simulink model "car_park_simulation"  (R2023b)
settings: Solver=VariableStepAuto  StartTime=0.0  StopTime=inf  RelTol=1e-3
libraries: simulink_extras x8, simulink x2
settings Model: Creator=abdul  LastModifiedBy=abdul

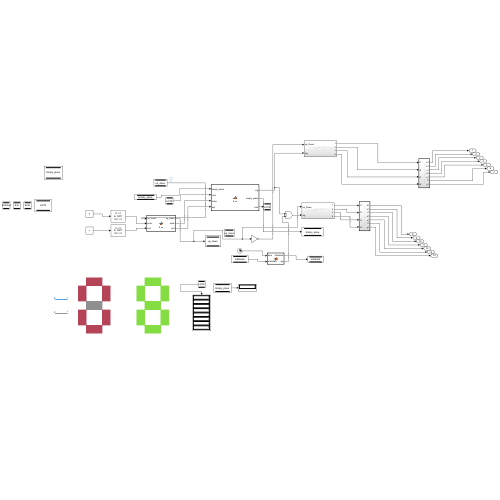
[thumbnail: Simulink's stored preview of the top-level diagram]
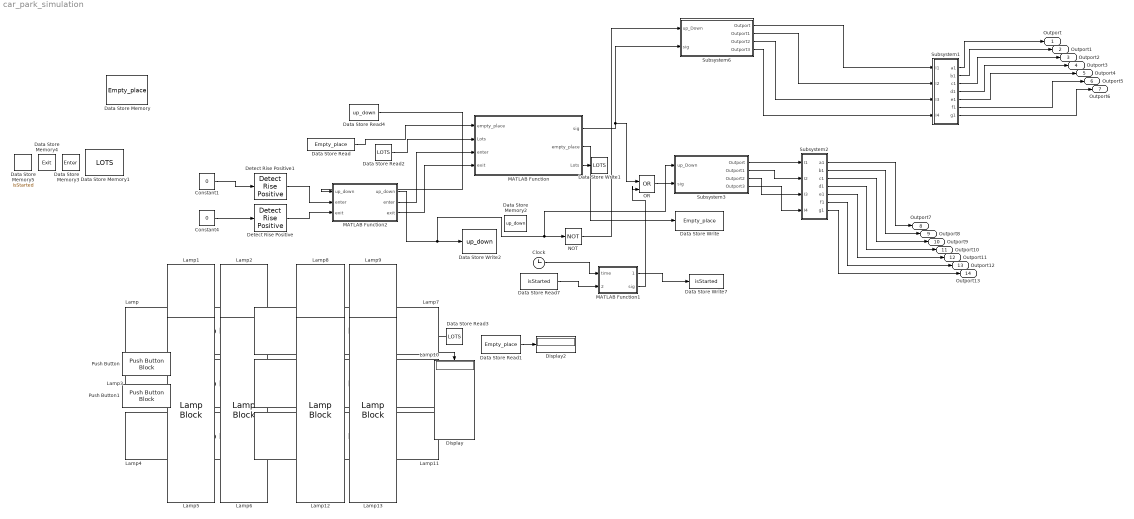
== system car_park_simulation ==
  Clock : Clock
  Constant1 : Constant  Value=0
  Constant4 : Constant  Value=0
  Data Store Memory : DataStoreMemory  DataStoreName=Empty_place  WriteAfterWriteMsg=warning  InitialValue=8  ShowAdditionalParam=off  OutDataTypeStr=double
  Data Store Memory1 : DataStoreMemory  DataStoreName=LOTS  WriteAfterWriteMsg=warning  InitialValue=[0,0,0,0,0,0,0,0]  ShowAdditionalParam=off
  Data Store Memory2 : DataStoreMemory  DataStoreName=up_down  WriteAfterWriteMsg=warning  ShowAdditionalParam=off
  Data Store Memory3 : DataStoreMemory  DataStoreName=Enter  WriteAfterWriteMsg=warning  ShowAdditionalParam=off
  Data Store Memory4 : DataStoreMemory  DataStoreName=Exit  WriteAfterWriteMsg=warning  ShowAdditionalParam=off
  Data Store Memory5 : DataStoreMemory  DataStoreName=isStarted  WriteAfterWriteMsg=warning  ShowAdditionalParam=off
  Data Store Read : DataStoreRead  DataStoreName=Empty_place  IndexOptions=Index vector (dialog)  Indices=1  OutputSizes=1
  Data Store Read1 : DataStoreRead  DataStoreName=Empty_place  IndexOptions=Index vector (dialog)  Indices=1  OutputSizes=1
  Data Store Read2 : DataStoreRead  DataStoreName=LOTS  IndexOptions=Index vector (dialog)  Indices=1  OutputSizes=1
  Data Store Read3 : DataStoreRead  DataStoreName=LOTS  IndexOptions=Index vector (dialog)  Indices=1  OutputSizes=1
  Data Store Read4 : DataStoreRead  DataStoreName=up_down  IndexOptions=Index vector (dialog)  Indices=1  OutputSizes=1
  Data Store Read7 : DataStoreRead  DataStoreName=isStarted  IndexOptions=Index vector (dialog)  Indices=1  OutputSizes=1
  Data Store Write : DataStoreWrite  DataStoreName=Empty_place  IndexOptions=Index vector (dialog)  Indices=1  OutputSizes=1
  Data Store Write1 : DataStoreWrite  DataStoreName=LOTS  IndexOptions=Index vector (dialog)  Indices=1  OutputSizes=1
  Data Store Write2 : DataStoreWrite  DataStoreName=up_down  IndexOptions=Index vector (dialog)  Indices=1  OutputSizes=1
  Data Store Write7 : DataStoreWrite  DataStoreName=isStarted  IndexOptions=Index vector (dialog)  Indices=1  OutputSizes=1
  Detect Rise Positive : simulink/Logic and Bit Operations/Detect Rise Positive  vinit=0  OutDataTypeStr=boolean
  Detect Rise Positive1 : simulink/Logic and Bit Operations/Detect Rise Positive  vinit=0  OutDataTypeStr=boolean
  Display : Display
  Display2 : Display
  Lamp{,1..13} (14 alike) : LampBlock  LabelPosition=Hide  Icon=Rectangle
  MATLAB Function : MATLAB Function  TreatAsAtomicUnit=on
  MATLAB Function1 : MATLAB Function  TreatAsAtomicUnit=on
  MATLAB Function2 : MATLAB Function  TreatAsAtomicUnit=on
  NOT : Logic  Operator=NOT  IconShape=distinctive  AllPortsSameDT=off  OutDataTypeStr=boolean
  OR : Logic  Operator=OR  IconShape=distinctive  AllPortsSameDT=off  OutDataTypeStr=boolean
  Push Button : PushButtonBlock  ButtonText=Exit  OffValue=0.000000
  Push Button1 : PushButtonBlock  ButtonText=Enter  OffValue=0.000000
  Subsystem1 : Subsystem  TreatAsAtomicUnit=on
  Subsystem2 : Subsystem  TreatAsAtomicUnit=on
  Subsystem3 : Subsystem
  Subsystem6 : Subsystem
  Outport : Outport
  Outport1 : Outport  Port=2
  Outport2 : Outport  Port=3
  Outport3 : Outport  Port=4
  Outport4 : Outport  Port=5
  Outport5 : Outport  Port=6
  Outport6 : Outport  Port=7
  Outport7 : Outport  Port=8
  Outport8 : Outport  Port=9
  Outport9 : Outport  Port=10
  Outport10 : Outport  Port=11
  Outport11 : Outport  Port=12
  Outport12 : Outport  Port=13
  Outport13 : Outport  Port=14
  wires:
  Data Store Read4/1 -> MATLAB Function2/1("up_down ")
  MATLAB Function2/3(exit) -> MATLAB Function/4(exit)
  Detect Rise Positive1/1 -> MATLAB Function2/2("enter ")
  MATLAB Function1/1(isStarted) -> Data Store Write7/1
  OR/1 -> Subsystem3/2(sig)
  MATLAB Function1/2(sig) -> OR/2
  Subsystem3/2(Outport1) -> Subsystem2/2(I2)
  MATLAB Function2/1(up_down) -> Subsystem3/1(up_Down), NOT/1, Data Store Write2/1
  Constant4/1 -> Detect Rise Positive/1
  Clock/1 -> MATLAB Function1/1(time)
  Subsystem6/2(Outport1) -> Subsystem1/2(I2)
  Subsystem2/3(c1) -> Outport9/1
  Subsystem2/4(d1) -> Outport10/1
  Subsystem6/4(Outport3) -> Subsystem1/4(I4)
  Constant1/1 -> Detect Rise Positive1/1
  Subsystem2/1(a1) -> Outport7/1
  Subsystem3/3(Outport2) -> Subsystem2/3(I3)
  Subsystem1/2(b1) -> Outport1/1
  Subsystem2/6(f1) -> Outport12/1
  Subsystem2/5(e1) -> Outport11/1
  Subsystem2/7(g1) -> Outport13/1
  MATLAB Function2/2(enter) -> MATLAB Function/3(enter)
  Subsystem1/3(c1) -> Outport2/1
  Subsystem1/5(e1) -> Outport4/1
  Subsystem1/1(a1) -> Outport/1
  Subsystem1/7(g1) -> Outport6/1
  Subsystem1/4(d1) -> Outport3/1
  Data Store Read7/1 -> MATLAB Function1/2("isStarted ")
  Subsystem2/2(b1) -> Outport8/1
  Subsystem6/3(Outport2) -> Subsystem1/3(I3)
  Data Store Read1/1 -> Display2/1
  MATLAB Function/3(Lots) -> Data Store Write1/1
  Subsystem1/6(f1) -> Outport5/1
  Data Store Read/1 -> MATLAB Function/1("empty_place ")
  Data Store Read3/1 -> Display/1
  Data Store Read2/1 -> MATLAB Function/2("Lots ")
  Subsystem3/1(Outport) -> Subsystem2/1(I1)
  Subsystem3/4(Outport3) -> Subsystem2/4(I4)
  Subsystem6/1(Outport) -> Subsystem1/1(I1)
  MATLAB Function/1(sig) -> Subsystem6/2(sig), OR/1
  Detect Rise Positive/1 -> MATLAB Function2/3("exit ")
  MATLAB Function/2(empty_place) -> Data Store Write/1
  NOT/1 -> Subsystem6/1(up_Down)

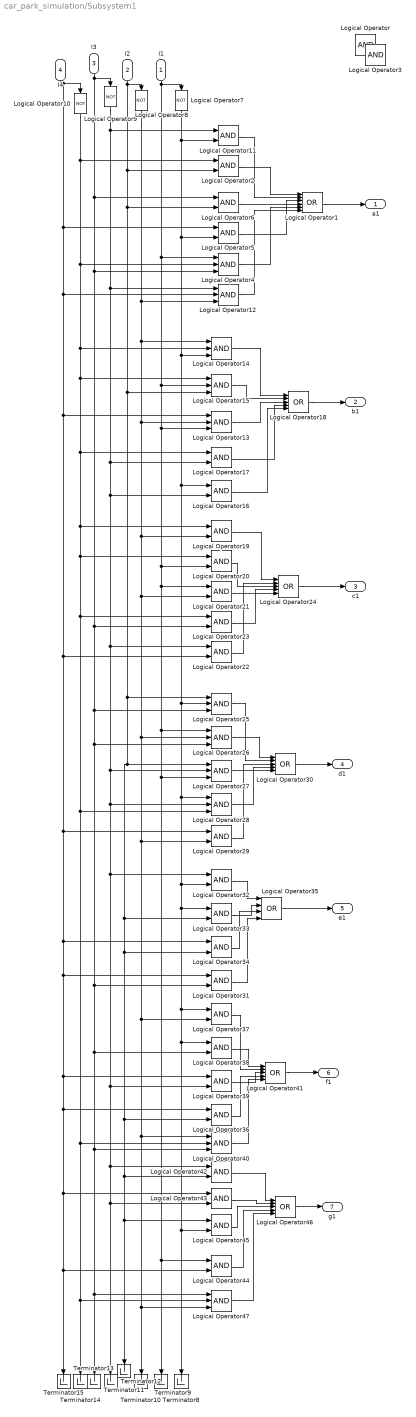
== system car_park_simulation/Subsystem1 ==
  I1 : Inport
  I2 : Inport  Port=2
  I3 : Inport  Port=3
  I4 : Inport  Port=4
  Logical Operator{,2..3,5..6,11,16..17,19..23,29,31..34,36..39,42..45} (26 alike) : Logic  AllPortsSameDT=off  OutDataTypeStr=boolean
  Logical Operator1 : Logic  Operator=OR  Inputs=6  AllPortsSameDT=off  OutDataTypeStr=boolean
  Logical Operator{7..10} (4 alike) : Logic  Operator=NOT  AllPortsSameDT=off  OutDataTypeStr=boolean
  Logical Operator{4,12..15,25..28,40,47} (11 alike) : Logic  Inputs=3  AllPortsSameDT=off  OutDataTypeStr=boolean
  Logical Operator{18,24,30,41,46} (5 alike) : Logic  Operator=OR  Inputs=5  AllPortsSameDT=off  OutDataTypeStr=boolean
  Logical Operator35 : Logic  Operator=OR  Inputs=4  AllPortsSameDT=off  OutDataTypeStr=boolean
  Terminator{8..15} (8 alike) : Terminator
  a1 : Outport
  b1 : Outport  Port=2
  c1 : Outport  Port=3
  d1 : Outport  Port=4
  e1 : Outport  Port=5
  f1 : Outport  Port=6
  g1 : Outport  Port=7
  wires:
  I1/1 -> Logical Operator7/1, Logical Operator4/1, Logical Operator26/1, Logical Operator27/3, Logical Operator44/1, Terminator9/1, Logical Operator21/1, Logical Operator20/2, Logical Operator13/3, Logical Operator15/2
  I4/1 -> Logical Operator5/1, Logical Operator12/2, Logical Operator29/1, Logical Operator31/1, Logical Operator39/1, Logical Operator43/1, Terminator15/1, Logical Operator44/2, Logical Operator36/1, Logical Operator34/1, Logical Operator22/2, Logical Operator13/1, Logical Operator10/1
  I3/1 -> Terminator13/1, Logical Operator47/1, Logical Operator40/3, Logical Operator38/2, Logical Operator31/2, Logical Operator26/3, Logical Operator25/3, Logical Operator23/2, Logical Operator4/3, Logical Operator6/1, Logical Operator9/1
  I2/1 -> Logical Operator15/3, Logical Operator33/2, Logical Operator45/1, Terminator11/1, Logical Operator42/2, Logical Operator36/2, Logical Operator34/2, Logical Operator27/1, Logical Operator25/1, Logical Operator6/2, Logical Operator2/2, Logical Operator8/1
  Logical Operator7/1 -> Logical Operator5/2, Logical Operator16/1, Logical Operator28/1, Logical Operator32/2, Logical Operator33/1, Logical Operator37/1, Logical Operator38/1, Terminator8/1, Logical Operator45/2, Logical Operator25/2, Logical Operator14/3, Logical Operator11/2
  Logical Operator8/1 -> Logical Operator14/1, Logical Operator21/2, Logical Operator26/2, Logical Operator40/1, Terminator10/1, Logical Operator47/3, Logical Operator37/2, Logical Operator29/2, Logical Operator19/2, Logical Operator13/2, Logical Operator12/3
  Logical Operator9/1 -> Logical Operator11/1, Logical Operator12/1, Logical Operator16/2, Logical Operator22/1, Logical Operator27/2, Logical Operator28/2, Terminator12/1, Logical Operator43/2, Logical Operator42/1, Logical Operator39/2, Logical Operator32/1, Logical Operator17/2
  Logical Operator10/1 -> Logical Operator2/1, Logical Operator4/2, Logical Operator14/2, Logical Operator15/1, Logical Operator28/3, Logical Operator40/2, Logical Operator47/2, Terminator14/1, Logical Operator23/1, Logical Operator20/1, Logical Operator19/1, Logical Operator17/1
  Logical Operator6/1 -> Logical Operator1/4
  Logical Operator4/1 -> Logical Operator1/5
  Logical Operator12/1 -> Logical Operator1/6
  Logical Operator5/1 -> Logical Operator1/3
  Logical Operator2/1 -> Logical Operator1/1
  Logical Operator11/1 -> Logical Operator1/2
  Logical Operator1/1 -> a1/1
  Logical Operator14/1 -> Logical Operator18/1
  Logical Operator15/1 -> Logical Operator18/2
  Logical Operator13/1 -> Logical Operator18/3
  Logical Operator17/1 -> Logical Operator18/4
  Logical Operator16/1 -> Logical Operator18/5
  Logical Operator18/1 -> b1/1
  Logical Operator21/1 -> Logical Operator24/5
  Logical Operator23/1 -> Logical Operator24/4
  Logical Operator22/1 -> Logical Operator24/2
  Logical Operator20/1 -> Logical Operator24/3
  Logical Operator19/1 -> Logical Operator24/1
  Logical Operator24/1 -> c1/1
  Logical Operator27/1 -> Logical Operator30/5
  Logical Operator28/1 -> Logical Operator30/4
  Logical Operator29/1 -> Logical Operator30/3
  Logical Operator26/1 -> Logical Operator30/1
  Logical Operator25/1 -> Logical Operator30/2
  Logical Operator30/1 -> d1/1
  Logical Operator31/1 -> Logical Operator35/4
  Logical Operator34/1 -> Logical Operator35/3
  Logical Operator33/1 -> Logical Operator35/2
  Logical Operator32/1 -> Logical Operator35/1
  Logical Operator35/1 -> e1/1
  Logical Operator40/1 -> Logical Operator41/5
  Logical Operator36/1 -> Logical Operator41/4
  Logical Operator39/1 -> Logical Operator41/3
  Logical Operator38/1 -> Logical Operator41/1
  Logical Operator37/1 -> Logical Operator41/2
  Logical Operator41/1 -> f1/1
  Logical Operator46/1 -> g1/1
  Logical Operator47/1 -> Logical Operator46/5
  Logical Operator44/1 -> Logical Operator46/4
  Logical Operator45/1 -> Logical Operator46/3
  Logical Operator43/1 -> Logical Operator46/2
  Logical Operator42/1 -> Logical Operator46/1

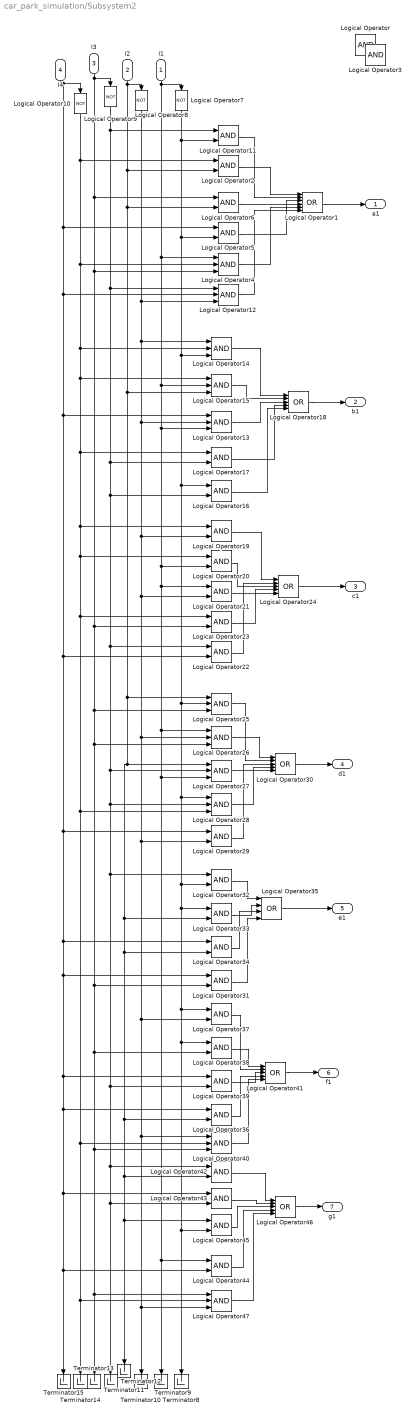
== system car_park_simulation/Subsystem2 ==
  I1 : Inport
  I2 : Inport  Port=2
  I3 : Inport  Port=3
  I4 : Inport  Port=4
  Logical Operator{,2..3,5..6,11,16..17,19..23,29,31..34,36..39,42..45} (26 alike) : Logic  AllPortsSameDT=off  OutDataTypeStr=boolean
  Logical Operator1 : Logic  Operator=OR  Inputs=6  AllPortsSameDT=off  OutDataTypeStr=boolean
  Logical Operator{7..10} (4 alike) : Logic  Operator=NOT  AllPortsSameDT=off  OutDataTypeStr=boolean
  Logical Operator{4,12..15,25..28,40,47} (11 alike) : Logic  Inputs=3  AllPortsSameDT=off  OutDataTypeStr=boolean
  Logical Operator{18,24,30,41,46} (5 alike) : Logic  Operator=OR  Inputs=5  AllPortsSameDT=off  OutDataTypeStr=boolean
  Logical Operator35 : Logic  Operator=OR  Inputs=4  AllPortsSameDT=off  OutDataTypeStr=boolean
  Terminator{8..15} (8 alike) : Terminator
  a1 : Outport
  b1 : Outport  Port=2
  c1 : Outport  Port=3
  d1 : Outport  Port=4
  e1 : Outport  Port=5
  f1 : Outport  Port=6
  g1 : Outport  Port=7
  wires:
  I1/1 -> Logical Operator7/1, Logical Operator4/1, Logical Operator26/1, Logical Operator27/3, Logical Operator44/1, Terminator9/1, Logical Operator21/1, Logical Operator20/2, Logical Operator13/3, Logical Operator15/2
  I4/1 -> Logical Operator5/1, Logical Operator12/2, Logical Operator29/1, Logical Operator31/1, Logical Operator39/1, Logical Operator43/1, Terminator15/1, Logical Operator44/2, Logical Operator36/1, Logical Operator34/1, Logical Operator22/2, Logical Operator13/1, Logical Operator10/1
  I3/1 -> Terminator13/1, Logical Operator47/1, Logical Operator40/3, Logical Operator38/2, Logical Operator31/2, Logical Operator26/3, Logical Operator25/3, Logical Operator23/2, Logical Operator4/3, Logical Operator6/1, Logical Operator9/1
  I2/1 -> Logical Operator15/3, Logical Operator33/2, Logical Operator45/1, Terminator11/1, Logical Operator42/2, Logical Operator36/2, Logical Operator34/2, Logical Operator27/1, Logical Operator25/1, Logical Operator6/2, Logical Operator2/2, Logical Operator8/1
  Logical Operator7/1 -> Logical Operator5/2, Logical Operator16/1, Logical Operator28/1, Logical Operator32/2, Logical Operator33/1, Logical Operator37/1, Logical Operator38/1, Terminator8/1, Logical Operator45/2, Logical Operator25/2, Logical Operator14/3, Logical Operator11/2
  Logical Operator8/1 -> Logical Operator14/1, Logical Operator21/2, Logical Operator26/2, Logical Operator40/1, Terminator10/1, Logical Operator47/3, Logical Operator37/2, Logical Operator29/2, Logical Operator19/2, Logical Operator13/2, Logical Operator12/3
  Logical Operator9/1 -> Logical Operator11/1, Logical Operator12/1, Logical Operator16/2, Logical Operator22/1, Logical Operator27/2, Logical Operator28/2, Terminator12/1, Logical Operator43/2, Logical Operator42/1, Logical Operator39/2, Logical Operator32/1, Logical Operator17/2
  Logical Operator10/1 -> Logical Operator2/1, Logical Operator4/2, Logical Operator14/2, Logical Operator15/1, Logical Operator28/3, Logical Operator40/2, Logical Operator47/2, Terminator14/1, Logical Operator23/1, Logical Operator20/1, Logical Operator19/1, Logical Operator17/1
  Logical Operator6/1 -> Logical Operator1/4
  Logical Operator4/1 -> Logical Operator1/5
  Logical Operator12/1 -> Logical Operator1/6
  Logical Operator5/1 -> Logical Operator1/3
  Logical Operator2/1 -> Logical Operator1/1
  Logical Operator11/1 -> Logical Operator1/2
  Logical Operator1/1 -> a1/1
  Logical Operator14/1 -> Logical Operator18/1
  Logical Operator15/1 -> Logical Operator18/2
  Logical Operator13/1 -> Logical Operator18/3
  Logical Operator17/1 -> Logical Operator18/4
  Logical Operator16/1 -> Logical Operator18/5
  Logical Operator18/1 -> b1/1
  Logical Operator21/1 -> Logical Operator24/5
  Logical Operator23/1 -> Logical Operator24/4
  Logical Operator22/1 -> Logical Operator24/2
  Logical Operator20/1 -> Logical Operator24/3
  Logical Operator19/1 -> Logical Operator24/1
  Logical Operator24/1 -> c1/1
  Logical Operator27/1 -> Logical Operator30/5
  Logical Operator28/1 -> Logical Operator30/4
  Logical Operator29/1 -> Logical Operator30/3
  Logical Operator26/1 -> Logical Operator30/1
  Logical Operator25/1 -> Logical Operator30/2
  Logical Operator30/1 -> d1/1
  Logical Operator31/1 -> Logical Operator35/4
  Logical Operator34/1 -> Logical Operator35/3
  Logical Operator33/1 -> Logical Operator35/2
  Logical Operator32/1 -> Logical Operator35/1
  Logical Operator35/1 -> e1/1
  Logical Operator40/1 -> Logical Operator41/5
  Logical Operator36/1 -> Logical Operator41/4
  Logical Operator39/1 -> Logical Operator41/3
  Logical Operator38/1 -> Logical Operator41/1
  Logical Operator37/1 -> Logical Operator41/2
  Logical Operator41/1 -> f1/1
  Logical Operator46/1 -> g1/1
  Logical Operator47/1 -> Logical Operator46/5
  Logical Operator44/1 -> Logical Operator46/4
  Logical Operator45/1 -> Logical Operator46/3
  Logical Operator43/1 -> Logical Operator46/2
  Logical Operator42/1 -> Logical Operator46/1

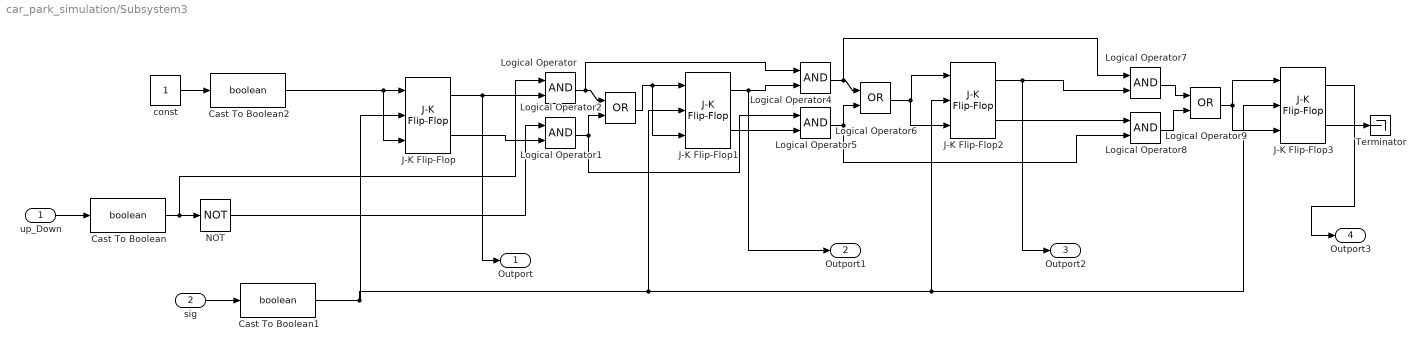
== system car_park_simulation/Subsystem3 ==
  up_Down : Inport
  sig : Inport  Port=2
  Cast To Boolean : DataTypeConversion  OutDataTypeStr=boolean  SaturateOnIntegerOverflow=off  RndMeth=Floor
  Cast To Boolean1 : DataTypeConversion  OutDataTypeStr=boolean  SaturateOnIntegerOverflow=off  RndMeth=Floor
  Cast To Boolean2 : DataTypeConversion  OutDataTypeStr=boolean  SaturateOnIntegerOverflow=off  RndMeth=Floor
  J-K Flip-Flop{,1..3} (4 alike) : simulink_extras/Flip Flops/J-K Flip-Flop  initial_condition=0
  Logical Operator{,1,4..5,7..8} (6 alike) : Logic  AllPortsSameDT=off  OutDataTypeStr=boolean
  Logical Operator2 : Logic  Operator=OR  AllPortsSameDT=off  OutDataTypeStr=boolean
  Logical Operator6 : Logic  Operator=OR  AllPortsSameDT=off  OutDataTypeStr=boolean
  Logical Operator9 : Logic  Operator=OR  AllPortsSameDT=off  OutDataTypeStr=boolean
  NOT : Logic  Operator=NOT  IconShape=distinctive  AllPortsSameDT=off  OutDataTypeStr=boolean
  Terminator : Terminator
  const : Constant  SampleTime=-1
  Outport : Outport
  Outport1 : Outport  Port=2
  Outport2 : Outport  Port=3
  Outport3 : Outport  Port=4
  wires:
  J-K Flip-Flop3/1 -> Outport3/1
  J-K Flip-Flop3/2 -> Terminator/1
  J-K Flip-Flop2/1 -> Logical Operator7/2, Outport2/1
  J-K Flip-Flop1/2 -> Logical Operator5/2
  J-K Flip-Flop1/1 -> Logical Operator4/2, Outport1/1
  Cast To Boolean2/1 -> J-K Flip-Flop/1, J-K Flip-Flop/3
  const/1 -> Cast To Boolean2/1
  J-K Flip-Flop2/2 -> Logical Operator8/1
  Logical Operator7/1 -> Logical Operator9/1
  Logical Operator8/1 -> Logical Operator9/2
  Logical Operator4/1 -> Logical Operator7/1, Logical Operator6/1
  Logical Operator5/1 -> Logical Operator6/2, Logical Operator8/2
  Cast To Boolean1/1 -> J-K Flip-Flop3/2, J-K Flip-Flop2/2, J-K Flip-Flop1/2, J-K Flip-Flop/2
  sig/1 -> Cast To Boolean1/1
  Cast To Boolean/1 -> Logical Operator/1, NOT/1
  up_Down/1 -> Cast To Boolean/1
  J-K Flip-Flop/1 -> Logical Operator/2, Outport/1
  J-K Flip-Flop/2 -> Logical Operator1/2
  Logical Operator1/1 -> Logical Operator2/2, Logical Operator5/1
  Logical Operator/1 -> Logical Operator4/1, Logical Operator2/1
  Logical Operator2/1 -> J-K Flip-Flop1/3, J-K Flip-Flop1/1
  Logical Operator9/1 -> J-K Flip-Flop3/1, J-K Flip-Flop3/3
  Logical Operator6/1 -> J-K Flip-Flop2/3, J-K Flip-Flop2/1
  NOT/1 -> Logical Operator1/1

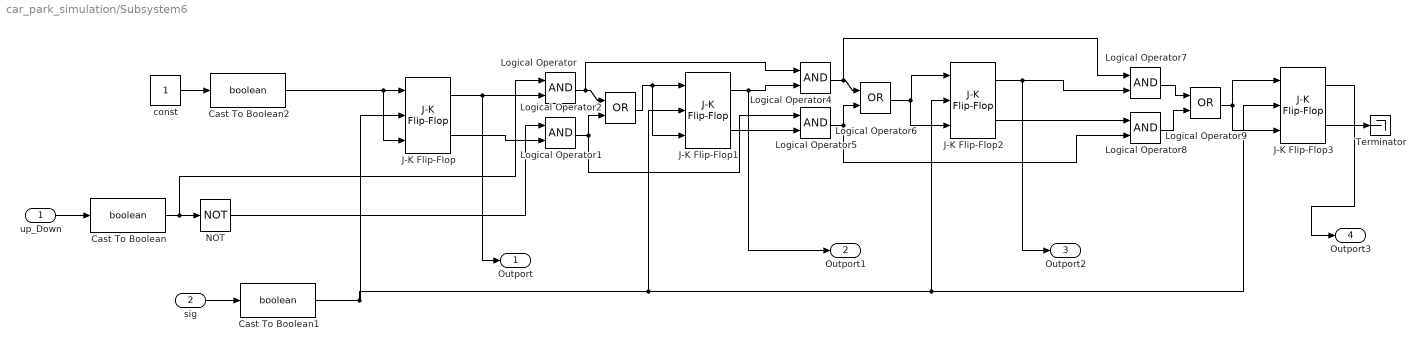
== system car_park_simulation/Subsystem6 ==
  up_Down : Inport
  sig : Inport  Port=2
  Cast To Boolean : DataTypeConversion  OutDataTypeStr=boolean  SaturateOnIntegerOverflow=off  RndMeth=Floor
  Cast To Boolean1 : DataTypeConversion  OutDataTypeStr=boolean  SaturateOnIntegerOverflow=off  RndMeth=Floor
  Cast To Boolean2 : DataTypeConversion  OutDataTypeStr=boolean  SaturateOnIntegerOverflow=off  RndMeth=Floor
  J-K Flip-Flop{,1..3} (4 alike) : simulink_extras/Flip Flops/J-K Flip-Flop  initial_condition=0
  Logical Operator{,1,4..5,7..8} (6 alike) : Logic  AllPortsSameDT=off  OutDataTypeStr=boolean
  Logical Operator2 : Logic  Operator=OR  AllPortsSameDT=off  OutDataTypeStr=boolean
  Logical Operator6 : Logic  Operator=OR  AllPortsSameDT=off  OutDataTypeStr=boolean
  Logical Operator9 : Logic  Operator=OR  AllPortsSameDT=off  OutDataTypeStr=boolean
  NOT : Logic  Operator=NOT  IconShape=distinctive  AllPortsSameDT=off  OutDataTypeStr=boolean
  Terminator : Terminator
  const : Constant  SampleTime=-1
  Outport : Outport
  Outport1 : Outport  Port=2
  Outport2 : Outport  Port=3
  Outport3 : Outport  Port=4
  wires:
  J-K Flip-Flop3/1 -> Outport3/1
  J-K Flip-Flop3/2 -> Terminator/1
  J-K Flip-Flop2/1 -> Logical Operator7/2, Outport2/1
  J-K Flip-Flop1/2 -> Logical Operator5/2
  J-K Flip-Flop1/1 -> Logical Operator4/2, Outport1/1
  Cast To Boolean2/1 -> J-K Flip-Flop/1, J-K Flip-Flop/3
  const/1 -> Cast To Boolean2/1
  J-K Flip-Flop2/2 -> Logical Operator8/1
  Logical Operator7/1 -> Logical Operator9/1
  Logical Operator8/1 -> Logical Operator9/2
  Logical Operator4/1 -> Logical Operator7/1, Logical Operator6/1
  Logical Operator5/1 -> Logical Operator6/2, Logical Operator8/2
  Cast To Boolean1/1 -> J-K Flip-Flop3/2, J-K Flip-Flop2/2, J-K Flip-Flop1/2, J-K Flip-Flop/2
  sig/1 -> Cast To Boolean1/1
  Cast To Boolean/1 -> Logical Operator/1, NOT/1
  up_Down/1 -> Cast To Boolean/1
  J-K Flip-Flop/1 -> Logical Operator/2, Outport/1
  J-K Flip-Flop/2 -> Logical Operator1/2
  Logical Operator1/1 -> Logical Operator2/2, Logical Operator5/1
  Logical Operator/1 -> Logical Operator4/1, Logical Operator2/1
  Logical Operator2/1 -> J-K Flip-Flop1/3, J-K Flip-Flop1/1
  Logical Operator9/1 -> J-K Flip-Flop3/1, J-K Flip-Flop3/3
  Logical Operator6/1 -> J-K Flip-Flop2/3, J-K Flip-Flop2/1
  NOT/1 -> Logical Operator1/1

== matlab function car_park_simulation/MATLAB Function1 ==
  data: time input; isStarted input; isStarted output; sig output
function [isStarted,sig] = fcn(time, isStarted)
sig=0;
if(mod(time,1000)==0)
    if(isStarted<8)
        sig=1;
        isStarted=isStarted+1;
    else
        sig=0;
    end
end

== matlab function car_park_simulation/MATLAB Function ==
  data: empty_place input; Lots input; enter input; exit input; sig output; empty_place output; Lots output
function [sig,empty_place,Lots] = fcn(empty_place,Lots,enter,exit)
sig=0;

if(enter>0 && empty_place>0)

    for i=1:1:8
        if(Lots(i)==0)
            empty_place=empty_place-1;
            Lots(i)=1;
            break
        end
    end
    sig=1;
end

if(exit>0 && empty_place<8)


    
    for i=1:length(Lots)
        if(Lots(i)==1)
            empty_place=empty_place+1;
            Lots(i)=0;
            break
        end
    end
    sig=1;
end

== matlab function car_park_simulation/MATLAB Function2 ==
  data: up_down input; enter input; up_down output; exit input; enter output; exit output
function [up_down,enter,exit] = fcn(up_down,enter,exit)
if(enter>0)
    up_down=0;
end
if(exit>0)
    up_down=1;
end
